simulink library "Autonomous_lib"  (R2023b)
settings: Solver=VariableStepAuto  StartTime=0.0  StopTime=10.0  RelTol=1e-3
undefined symbols (not defined in the file): Spline_Num_Poses_default, Spline_Ref_Poses_default
settings Model: Creator=FIRSTMentor  LastModifiedBy=ander

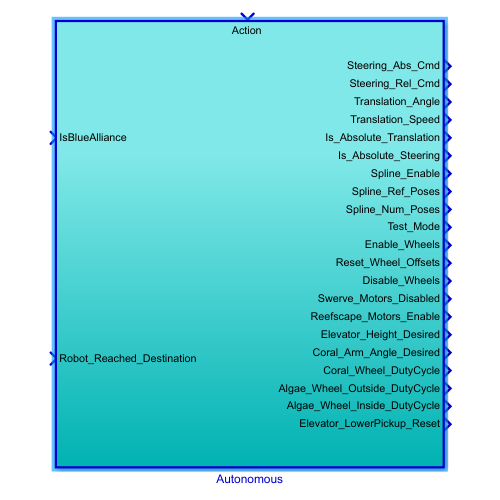
[thumbnail: Simulink's stored preview of the top-level diagram]
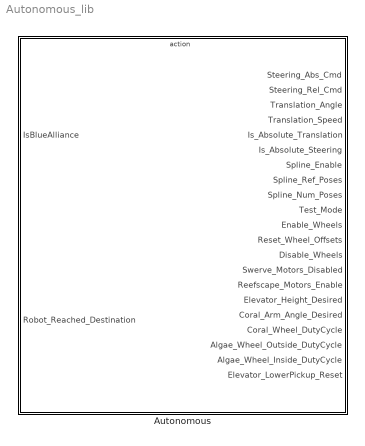
== system Autonomous_lib ==
  Autonomous : Subsystem  TreatAsAtomicUnit=on

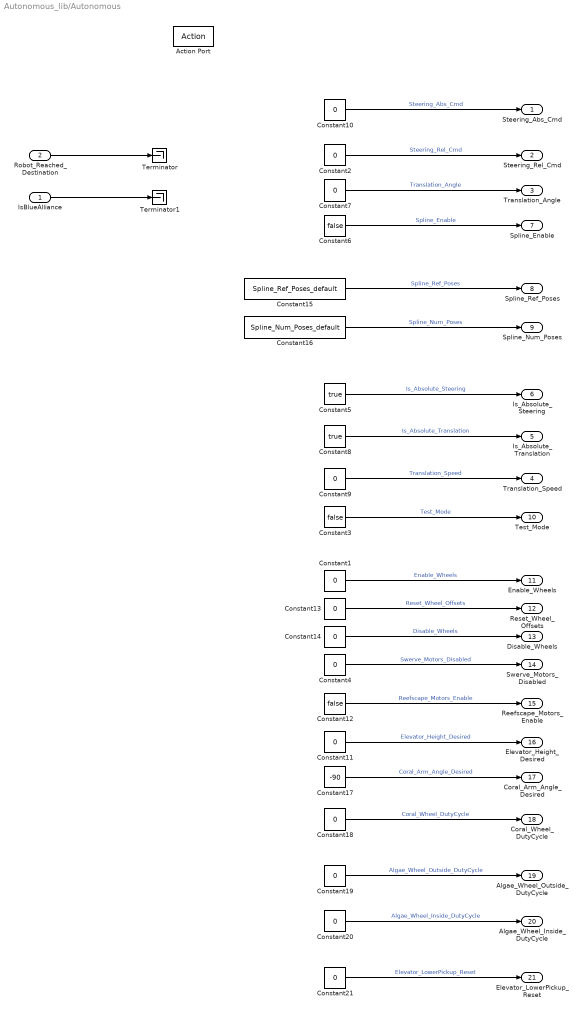
== system Autonomous_lib/Autonomous ==
  IsBlueAlliance : Inport
  Robot_Reached_Destination : Inport  Port=2
  Action Port : ActionPort  InitializeStates=reset
  Constant{1..2,7,9..11,13..14,18..20} (11 alike) : Constant  Value=0
  Constant12 : Constant  Value=false  OutDataTypeStr=boolean
  Constant15 : Constant  Value=Spline_Ref_Poses_default
  Constant16 : Constant  Value=Spline_Num_Poses_default  OutDataTypeStr=double
  Constant17 : Constant  Value=-90
  Constant21 : Constant  Value=0  OutDataTypeStr=boolean
  Constant3 : Constant  Value=false  OutDataTypeStr=boolean
  Constant4 : Constant  Value=0  OutDataTypeStr=boolean
  Constant5 : Constant  Value=true
  Constant6 : Constant  Value=false
  Constant8 : Constant  Value=true
  Terminator : Terminator
  Terminator1 : Terminator
  Steering_Abs_Cmd : Outport
  Steering_Rel_Cmd : Outport  Port=2
  Translation_Angle : Outport  Port=3
  Translation_Speed : Outport  Port=4
  Is_Absolute_Translation : Outport  Port=5
  Is_Absolute_Steering : Outport  Port=6
  Spline_Enable : Outport  Port=7
  Spline_Ref_Poses : Outport  Port=8
  Spline_Num_Poses : Outport  Port=9
  Test_Mode : Outport  Port=10
  Enable_Wheels : Outport  Port=11
  Reset_Wheel_Offsets : Outport  Port=12
  Disable_Wheels : Outport  Port=13
  Swerve_Motors_Disabled : Outport  Port=14
  Reefscape_Motors_Enable : Outport  Port=15
  Elevator_Height_Desired : Outport  Port=16
  Coral_Arm_Angle_Desired : Outport  Port=17
  Coral_Wheel_DutyCycle : Outport  Port=18
  Algae_Wheel_Outside_DutyCycle : Outport  Port=19
  Algae_Wheel_Inside_DutyCycle : Outport  Port=20
  Elevator_LowerPickup_Reset : Outport  Port=21
  wires:
  Constant2/1 -> Steering_Rel_Cmd/1  "Steering_Rel_Cmd"
  Constant15/1 -> Spline_Ref_Poses/1  "Spline_Ref_Poses"
  Constant7/1 -> Translation_Angle/1  "Translation_Angle"
  Constant3/1 -> Test_Mode/1  "Test_Mode"
  Constant14/1 -> Disable_Wheels/1  "Disable_Wheels"
  Constant13/1 -> Reset_Wheel_Offsets/1  "Reset_Wheel_Offsets"
  Constant4/1 -> Swerve_Motors_Disabled/1  "Swerve_Motors_Disabled"
  Constant1/1 -> Enable_Wheels/1  "Enable_Wheels"
  Robot_Reached_Destination/1 -> Terminator/1
  IsBlueAlliance/1 -> Terminator1/1
  Constant5/1 -> Is_Absolute_Steering/1  "Is_Absolute_Steering"
  Constant8/1 -> Is_Absolute_Translation/1  "Is_Absolute_Translation"
  Constant9/1 -> Translation_Speed/1  "Translation_Speed"
  Constant6/1 -> Spline_Enable/1  "Spline_Enable"
  Constant10/1 -> Steering_Abs_Cmd/1  "Steering_Abs_Cmd"
  Constant16/1 -> Spline_Num_Poses/1  "Spline_Num_Poses"
  Constant11/1 -> Elevator_Height_Desired/1  "Elevator_Height_Desired"
  Constant12/1 -> Reefscape_Motors_Enable/1  "Reefscape_Motors_Enable"
  Constant18/1 -> Coral_Wheel_DutyCycle/1  "Coral_Wheel_DutyCycle"
  Constant17/1 -> Coral_Arm_Angle_Desired/1  "Coral_Arm_Angle_Desired"
  Constant19/1 -> Algae_Wheel_Outside_DutyCycle/1  "Algae_Wheel_Outside_DutyCycle"
  Constant20/1 -> Algae_Wheel_Inside_DutyCycle/1  "Algae_Wheel_Inside_DutyCycle"
  Constant21/1 -> Elevator_LowerPickup_Reset/1  "Elevator_LowerPickup_Reset"
